simulink model "CruiseCtrl_StateFeedback"  (R2023b)
settings: Solver=ode45  StartTime=0.0  StopTime=40  MaxStep=0.01  RelTol=1e-3  EnableMultiTasking=on
values from neighbouring files (symbols this model uses):
  A = [-1.25, 0 ... (first row only)    [CruiseCtrl_StateFeedback_design.m]    (also in Driveline_ctrl_design.m = [ -ds/(Jf*r^2),  ds/(Jf*r), -cs/(Jf*r))
  alpha = 20*pi/180    (= 0.349065850399)    [CruiseCtrl_StateFeedback_design.m]
  B1 = [B H]    [CruiseCtrl_StateFeedback_design.m]    (also in Driveline_ctrl_design.m)
  C1 = eye(2)    [CruiseCtrl_StateFeedback_design.m]
  D1 = zeros(2)    [CruiseCtrl_StateFeedback_design.m]
  g = 9.82    [CruiseCtrl_StateFeedback_design.m]
  K = acker(A, B, polos_deseados)    [CruiseCtrl_StateFeedback_design.m]    (also in Driveline_ctrl_design.m = acker(A, B, [p1, p2, p3]))
  kr = -inv(C*inv(A-B*K)*B)    [CruiseCtrl_StateFeedback_design.m]    (also in Driveline_ctrl_design.m = -1 / (C_salida * ((A - B*K) \ B)))
  ue = rw*x1e/k/r    (= 0.214125)    [CruiseCtrl_StateFeedback_design.m]
  x1e = 0.5*rho*CD*Af*x2e^2+m*g*f    (= 3426)    [CruiseCtrl_StateFeedback_design.m]
  x2e = 20    [CruiseCtrl_StateFeedback_design.m]
settings Model: Creator=JonasMac  LastModifiedBy=tomas
settings SolverCC: AlgebraicLoopSolver=TrustRegion
settings DataIOCC: LimitDataPoints=on  SaveFormat=Array  ReturnWorkspaceOutputs=off
settings OptimizationCC: LifeSpan=inf
settings DebuggingCC: UnderspecifiedInitializationDetection=Classic  MergeDetectMultiDrivingBlocksExec=none  SolverPrmCheckMsg=warning  UnconnectedInputMsg=warning  UnconnectedOutputMsg=warning  UnconnectedLineMsg=warning  SFUnexpectedBacktrackingDiag=warning  SFNoUnconditionalDefaultTransitionDiag=warning  SFExecutionAtInitializationDiag=none  ArithmeticOperatorsInVariantConditions=warning
settings HardwareCC: ProdBitPerPointer=32  ProdBitPerSizeT=32  ProdBitPerPtrDiffT=32  ProdLargestAtomicFloat=None  ProdIntDivRoundTo=Undefined  ProdEndianess=Unspecified  ProdWordSize=32  ProdHWDeviceType=32-bit Generic
settings ModelReferenceCC: EnableRefExpFcnMdlSchedulingChecks=on  PropagateSignalLabelsOutOfModel=off
settings SFSimCC: SimUseLocalCustomCode=off  CustomCodeUndefinedFunction=UseInterfaceOnly
settings RTWCC: RTWUseLocalCustomCode=off
settings CodeAppCC: StateflowObjectComments=on
settings GRTTargetCC: TargetLangStandard=C89/C90 (ANSI)
settings ConfigComp: CovMetricSettings=dw  CovSaveCumulativeToWorkspaceVar=on  CovSaveSingleToWorkspaceVar=on  CovExternalEMLEnable=off

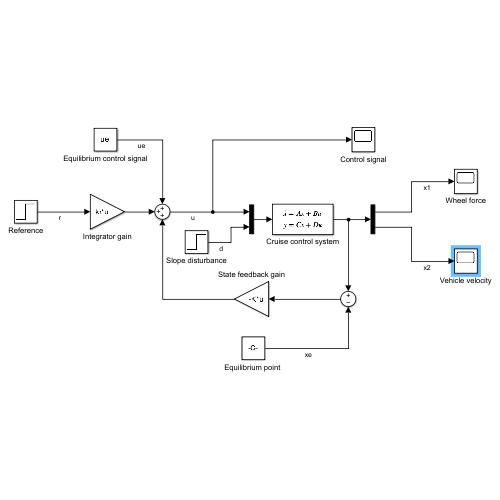
[thumbnail: Simulink's stored preview of the top-level diagram]
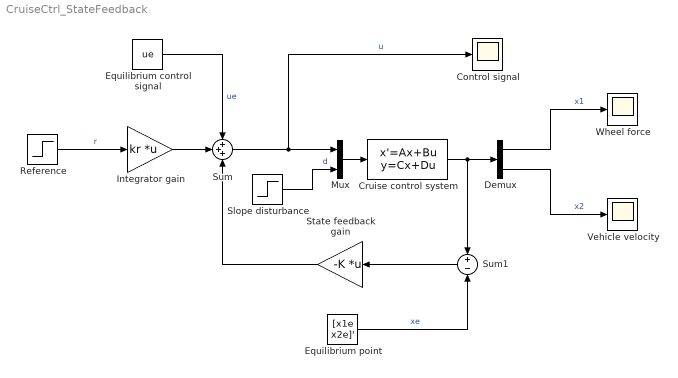
== system CruiseCtrl_StateFeedback ==
  Control signal : Scope
  Cruise control system : StateSpace  A=A  B=B1  C=C1  D=D1
  Demux : Demux  Outputs=2
  Equilibrium control signal : Constant  Value=ue
  "Equilibrium point " : Constant  Value=[x1e x2e]'
  Integrator gain : Gain  Gain=kr  Multiplication=Matrix(K*u)
  Mux : Mux  Inputs=2
  Reference : Step  After=5  SampleTime=0
  Slope disturbance : Step  Time=20  After=g*sin(alpha)  SampleTime=0
  State feedback gain : Gain  Gain=-K  Multiplication=Matrix(K*u)
  Sum : Sum  Inputs=+++
  Sum1 : Sum  Inputs=+-
  Vehicle velocity : Scope
  Wheel force : Scope
  wires:
  Demux/1 -> Wheel force/1  "x1"
  Demux/2 -> Vehicle velocity/1  "x2"
  Sum/1 -> Mux/1, Control signal/1  "u"
  Slope disturbance/1 -> Mux/2  "d"
  Integrator gain/1 -> Sum/2
  Equilibrium control signal/1 -> Sum/1  "ue"
  Cruise control system/1 -> Demux/1, Sum1/1
  Mux/1 -> Cruise control system/1
  State feedback gain/1 -> Sum/3
  Sum1/1 -> State feedback gain/1
  "Equilibrium point "/1 -> Sum1/2  "xe"
  Reference/1 -> Integrator gain/1  "r"
